simulink model "Prob1b"  (Simulink 7.0)
settings: Solver=ode45  StartTime=0.0  StopTime=30  RelTol=1e-8
settings Model: Creator=Kailu  LastModifiedBy=Kailu  ExtModeTrigMode=oneshot  ExtModeArmWhenConnect=off
settings DataIOCC: LimitDataPoints=off
settings OptimizationCC: BlockReduction=off  BooleanDataType=off
settings DebuggingCC: SaveWithParameterizedLinksMsg=none  SignalResolutionControl=TryResolveAllWithWarning  SolverPrmCheckMsg=none  MultiTaskDSMMsg=warning  MultiTaskCondExecSysMsg=none  StrictBusMsg=None
settings HardwareCC: TargetUnknown=on
settings RTWCC: IncludeERTFirstTime=on

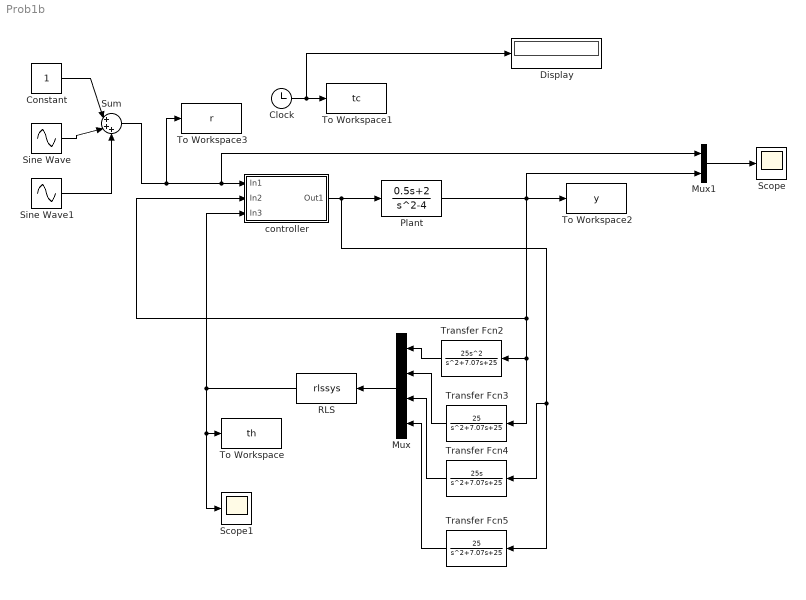
== system Prob1b ==
  Clock : Clock
      settings: Decimation=10
  Constant : Constant  OutDataType=sfix(16)  OutScaling=2^0
  Display : Display
  Mux : Mux  Orientation=left
  Mux1 : Mux  Inputs=2
  Plant : TransferFcn  Numerator=[ 0.5 2]  Denominator=[1 0 -4]
  RLS : S-Function  Orientation=left  FunctionName=rlssys  Parameters=[1;1;1],1000,2
  Scope : Scope
  Scope1 : Scope
  Sine Wave : Sin  SampleTime=0
  Sine Wave1 : Sin  Frequency=2  SampleTime=0
  Sum : Sum  Inputs=|+++  OutDataType=sfix(16)  OutScaling=2^0
  To Workspace : ToWorkspace  VariableName=th  SampleTime=0.01  SaveFormat=Array
  To Workspace1 : ToWorkspace  VariableName=tc  SampleTime=0.01  SaveFormat=Array
  To Workspace2 : ToWorkspace  VariableName=y  SampleTime=0.01  SaveFormat=Array
  To Workspace3 : ToWorkspace  VariableName=r  SampleTime=0.01  SaveFormat=Array
  Transfer Fcn2 : TransferFcn  Orientation=left  Numerator=[25 0 0]  Denominator=[1 7.07 25]
  Transfer Fcn3 : TransferFcn  Orientation=left  Numerator=[0 25]  Denominator=[1 7.07 25]
  Transfer Fcn4 : TransferFcn  Orientation=left  Numerator=[25 0]  Denominator=[1 7.07 25]
  Transfer Fcn5 : TransferFcn  Orientation=left  Numerator=[0 25]  Denominator=[1 7.07 25]
  controller : Subsystem
  wires:
  Clock/1 -> To Workspace1/1, Display/1
  Plant/1 -> To Workspace2/1, controller/2(In2), Transfer Fcn2/1, Transfer Fcn3/1, Mux1/2
  Sum/1 -> To Workspace3/1, controller/1(In1), Mux1/1
  controller/1(Out1) -> Plant/1, Transfer Fcn4/1, Transfer Fcn5/1
  Mux/1 -> RLS/1
  RLS/1 -> controller/3(In3), To Workspace/1, Scope1/1
  Transfer Fcn2/1 -> Mux/1
  Constant/1 -> Sum/1
  Sine Wave/1 -> Sum/2
  Sine Wave1/1 -> Sum/3
  Transfer Fcn3/1 -> Mux/2
  Transfer Fcn5/1 -> Mux/4
  Transfer Fcn4/1 -> Mux/3
  Mux1/1 -> Scope/1

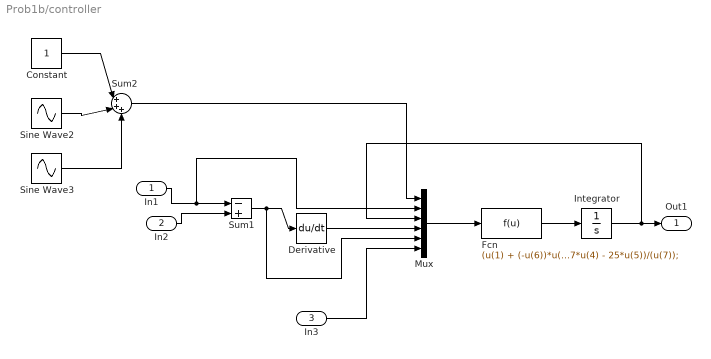
== system Prob1b/controller ==
  In1 : Inport
  In2 : Inport  Port=2
  In3 : Inport  Port=3
  Constant : Constant  OutDataType=sfix(16)  OutScaling=2^0
  Derivative : Derivative
  Fcn : Fcn  Expr=(u(1) + (-u(6))*u(2) - (u(8))*u(3) - 7.07*u(4) - 25*u(5))/(u(7));
  Integrator : Integrator
  Mux : Mux  Inputs=6
  Sine Wave2 : Sin  Amplitude=-1  SampleTime=0
  Sine Wave3 : Sin  Amplitude=-4  Frequency=2  SampleTime=0
  Sum1 : Sum  Inputs=-+  SaturateOnIntegerOverflow=on  InputSameDT=on
  Sum2 : Sum  Inputs=|+++  OutDataType=sfix(16)  OutScaling=2^0
  Out1 : Outport
  wires:
  In2/1 -> Sum1/2
  In1/1 -> Sum1/1, Mux/2
  Mux/1 -> Fcn/1
  Fcn/1 -> Integrator/1
  Derivative/1 -> Mux/4
  Constant/1 -> Sum2/1
  Sine Wave2/1 -> Sum2/2
  Sine Wave3/1 -> Sum2/3
  Sum2/1 -> Mux/1
  Sum1/1 -> Derivative/1, Mux/5
  In3/1 -> Mux/6
  Integrator/1 -> Out1/1, Mux/3
